simulink model "gm_VSD_and_Park_transformation_6Phase"  (R2022a)
settings: Solver=FixedStepDiscrete  StartTime=0.0  StopTime=0.2  RelTol=1e-3
libraries: hdlmdlgenlib x2
(part 1 of 2)
settings Model: Creator=Andre Merx  LastModifiedBy=Andre Merx
settings SolverCC: AlgebraicLoopSolver=TrustRegion
settings DataIOCC: LimitDataPoints=on  SaveOutput=off  SaveTime=off
settings OptimizationCC: BlockReduction=off  ConditionallyExecuteInputs=off  DefaultParameterBehavior=Inlined  InheritOutputTypeSmallerThanSingle=on  LifeSpan=inf
settings DebuggingCC: AlgebraicLoopMsg=error  InheritedTsInSrcMsg=none  SingleTaskRateTransMsg=error  UnconnectedInputMsg=warning  UnconnectedOutputMsg=warning  UnconnectedLineMsg=warning  AllowSymbolicDim=off  StrictBusMsg=ErrorOnBusTreatedAsVector  SFUnexpectedBacktrackingDiag=warning  SFNoUnconditionalDefaultTransitionDiag=warning  SFExecutionAtInitializationDiag=none  SFMachineParentedDataDiag=warning  ArithmeticOperatorsInVariantConditions=warning
settings HardwareCC: ProdBitPerPointer=32  ProdBitPerSizeT=32  ProdBitPerPtrDiffT=32  ProdLargestAtomicFloat=None  ProdIntDivRoundTo=Undefined  ProdEndianess=Unspecified  ProdWordSize=32  ProdHWDeviceType=ASIC/FPGA->ASIC/FPGA  ProdEqTarget=off
settings SFSimCC: SimUseLocalCustomCode=off  CustomCodeUndefinedFunction=UseInterfaceOnly
settings RTWCC: RTWUseLocalCustomCode=off
settings CodeAppCC: StateflowObjectComments=on
settings GRTTargetCC: TargetLangStandard=C89/C90 (ANSI)
settings ConfigComp: CovScope=ReferencedModels  CovMetricSettings=dw  CovSaveCumulativeToWorkspaceVar=on  CovSaveSingleToWorkspaceVar=on  CovExternalEMLEnable=off  CovSFcnEnable=off

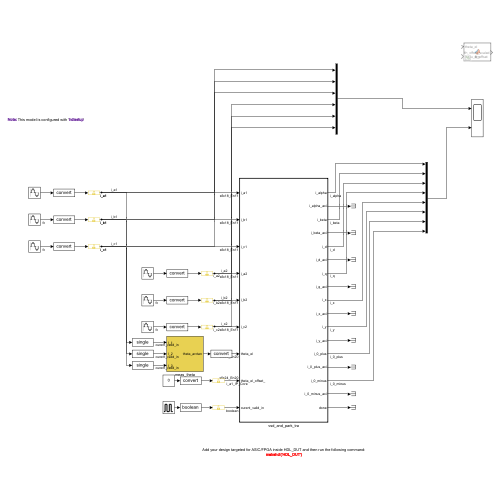
[thumbnail: Simulink's stored preview of the top-level diagram]
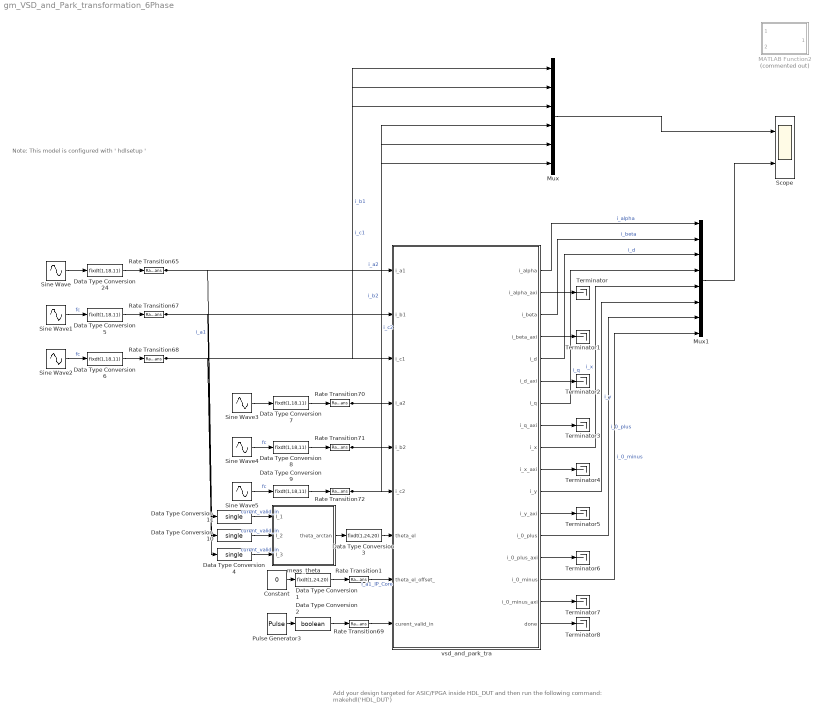
== system gm_VSD_and_Park_transformation_6Phase ==
  note: Add your design targeted for ASIC/FPGA inside HDL_DUT and then run the following command:
      | makehdl('HDL_DUT')
  note: Note: This model is configured with ' hdlsetup '
  Constant : Constant  Value=0  SampleTime=-1
  Data Type Conversion1 : DataTypeConversion  OutDataTypeStr=fixdt(1,24,20)  SaturateOnIntegerOverflow=off  RndMeth=Floor
  Data Type Conversion10 : DataTypeConversion  OutDataTypeStr=single  SaturateOnIntegerOverflow=off  RndMeth=Floor
  Data Type Conversion11 : DataTypeConversion  OutDataTypeStr=single  SaturateOnIntegerOverflow=off  RndMeth=Floor
  Data Type Conversion2 : DataTypeConversion  OutDataTypeStr=boolean  SaturateOnIntegerOverflow=off  RndMeth=Floor
  Data Type Conversion{5..9,24} (6 alike) : DataTypeConversion  OutDataTypeStr=fixdt(1,18,11)  SaturateOnIntegerOverflow=off  RndMeth=Floor
  Data Type Conversion3 : DataTypeConversion  OutDataTypeStr=fixdt(1,24,20)  SaturateOnIntegerOverflow=off  RndMeth=Floor
  Data Type Conversion4 : DataTypeConversion  OutDataTypeStr=single  SaturateOnIntegerOverflow=off  RndMeth=Floor
  MATLAB Function2 : MATLAB Function  Commented=on  TreatAsAtomicUnit=on
  Mux : Mux  Inputs=6
  Mux1 : Mux  Inputs=8
  Pulse Generator3 : DiscretePulseGenerator  PulseType=Time based  Period=1/100000  PulseWidth=5
  Rate Transition{1,65,67..72} (8 alike) : RateTransition  OutPortSampleTime=1.0000e-08
  Scope : Scope  NumInputPorts=2
  Sine Wave : Sin  Frequency=100  SampleTime=1/100000
  Sine Wave1 : Sin  Frequency=100  Phase=(4/3)*pi  SampleTime=1/100000
  Sine Wave2 : Sin  Frequency=100  Phase=(2/3)*pi  SampleTime=1/100000
  Sine Wave3 : Sin  Amplitude=0.5  Frequency=100  Phase=-pi/6  SampleTime=1/100000
  Sine Wave4 : Sin  Amplitude=0.5  Frequency=100  Phase=(7/6)*pi  SampleTime=1/100000
  Sine Wave5 : Sin  Amplitude=0.5  Frequency=100  Phase=(1/2)*pi  SampleTime=1/100000
  Terminator{,1..8} (9 alike) : Terminator
  meas_theta : Subsystem
  vsd_and_park_tra : Subsystem  TreatAsAtomicUnit=on
  wires:
  Data Type Conversion11/1 -> meas_theta/1(I_1)  "curent_valid_in"
  Data Type Conversion10/1 -> meas_theta/2(I_2)  "curent_valid_in"
  Data Type Conversion4/1 -> meas_theta/3(I_3)  "curent_valid_in"
  Data Type Conversion3/1 -> vsd_and_park_tra/7(theta_el)
  Mux1/1 -> Scope/2
  vsd_and_park_tra/15(i_0_minus) -> Mux1/8  "i_0_minus"
  vsd_and_park_tra/13(i_0_plus) -> Mux1/7  "i_0_plus"
  vsd_and_park_tra/11(i_y) -> Mux1/6  "i_y"
  vsd_and_park_tra/9(i_x) -> Mux1/5  "i_x"
  vsd_and_park_tra/7(i_q) -> Mux1/4  "i_q"
  vsd_and_park_tra/5(i_d) -> Mux1/3  "i_d"
  vsd_and_park_tra/3(i_beta) -> Mux1/2  "i_beta"
  vsd_and_park_tra/1(i_alpha) -> Mux1/1  "i_alpha"
  Mux/1 -> Scope/1
  vsd_and_park_tra/17(done) -> Terminator8/1
  vsd_and_park_tra/16(i_0_minus_axi) -> Terminator7/1
  vsd_and_park_tra/14(i_0_plus_axi) -> Terminator6/1
  vsd_and_park_tra/12(i_y_axi) -> Terminator5/1
  vsd_and_park_tra/10(i_x_axi) -> Terminator4/1
  vsd_and_park_tra/8(i_q_axi) -> Terminator3/1
  vsd_and_park_tra/6(i_d_axi) -> Terminator2/1
  vsd_and_park_tra/4(i_beta_axi) -> Terminator1/1
  vsd_and_park_tra/2(i_alpha_axi) -> Terminator/1
  Data Type Conversion2/1 -> Rate Transition69/1
  Rate Transition69/1 -> vsd_and_park_tra/9(curent_valid_in)
  Pulse Generator3/1 -> Data Type Conversion2/1
  Rate Transition1/1 -> vsd_and_park_tra/8(theta_el_offset_)  "i_a1_IP_Core"
  Data Type Conversion1/1 -> Rate Transition1/1
  Constant/1 -> Data Type Conversion1/1
  meas_theta/1(theta_arctan) -> Data Type Conversion3/1
  Rate Transition72/1 -> vsd_and_park_tra/6(i_c2), Mux/6  "i_c2"
  Rate Transition71/1 -> vsd_and_park_tra/5(i_b2), Mux/5  "i_b2"
  Rate Transition70/1 -> vsd_and_park_tra/4(i_a2), Mux/4  "i_a2"
  Data Type Conversion8/1 -> Rate Transition71/1
  Data Type Conversion7/1 -> Rate Transition70/1
  Sine Wave3/1 -> Data Type Conversion7/1
  Sine Wave4/1 -> Data Type Conversion8/1  "fc"
  Data Type Conversion9/1 -> Rate Transition72/1
  Sine Wave5/1 -> Data Type Conversion9/1  "fc"
  Rate Transition68/1 -> Data Type Conversion4/1, vsd_and_park_tra/3(i_c1), Mux/3  "i_c1"
  Rate Transition67/1 -> Data Type Conversion10/1, vsd_and_park_tra/2(i_b1), Mux/2  "i_b1"
  Rate Transition65/1 -> Data Type Conversion11/1, vsd_and_park_tra/1(i_a1), Mux/1  "i_a1"
  Data Type Conversion24/1 -> Rate Transition65/1
  Data Type Conversion5/1 -> Rate Transition67/1
  Sine Wave2/1 -> Data Type Conversion6/1  "fc"
  Data Type Conversion6/1 -> Rate Transition68/1
  Sine Wave1/1 -> Data Type Conversion5/1  "fc"
  Sine Wave/1 -> Data Type Conversion24/1

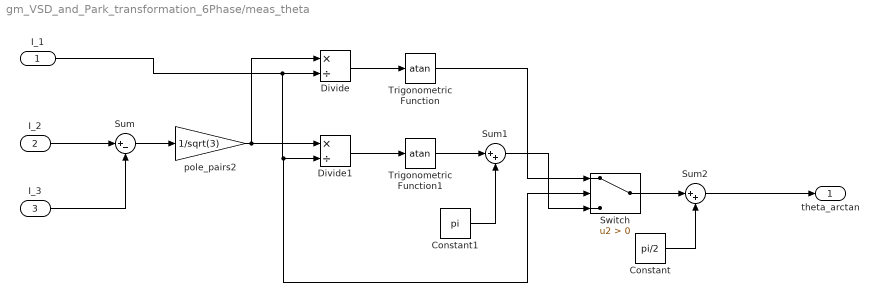
== system gm_VSD_and_Park_transformation_6Phase/meas_theta ==
  I_1 : Inport
  I_2 : Inport  Port=2
  I_3 : Inport  Port=3
  Constant : Constant  Value=pi/2
  Constant1 : Constant  Value=pi
  Divide : Product  Inputs=*/
  Divide1 : Product  Inputs=*/
  Sum : Sum  Inputs=|+-
  Sum1 : Sum  Inputs=|++
  Sum2 : Sum  Inputs=|++
  Switch : Switch  Criteria=u2 > Threshold  SaturateOnIntegerOverflow=off  InputSameDT=off
  Trigonometric Function : Trigonometry  Operator=atan
  Trigonometric Function1 : Trigonometry  Operator=atan
  pole_pairs2 : Gain  Gain=1/sqrt(3)
  theta_arctan : Outport  VectorParamsAs1DForOutWhenUnconnected=off
  wires:
  Sum2/1 -> theta_arctan/1
  Constant1/1 -> Sum1/2
  Constant/1 -> Sum2/2
  Switch/1 -> Sum2/1
  Trigonometric Function/1 -> Switch/1
  Sum1/1 -> Switch/3
  I_1/1 -> Divide/2, Divide1/2, Switch/2
  I_2/1 -> Sum/1
  I_3/1 -> Sum/2
  Sum/1 -> pole_pairs2/1
  pole_pairs2/1 -> Divide1/1, Divide/1
  Trigonometric Function1/1 -> Sum1/1
  Divide1/1 -> Trigonometric Function1/1
  Divide/1 -> Trigonometric Function/1

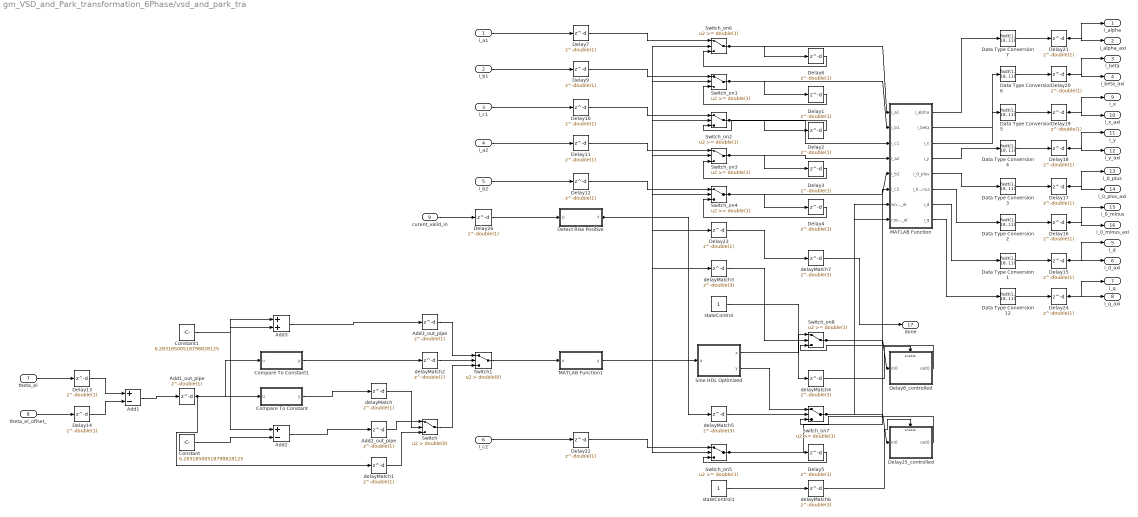
== system gm_VSD_and_Park_transformation_6Phase/vsd_and_park_tra ==
  i_a1 : Inport  OutDataTypeStr=fixdt(1, 18, 11)  PortDimensions=1  SampleTime=1e-08
  i_b1 : Inport  Port=2  OutDataTypeStr=fixdt(1, 18, 11)  PortDimensions=1  SampleTime=1e-08
  i_c1 : Inport  Port=3  OutDataTypeStr=fixdt(1, 18, 11)  PortDimensions=1  SampleTime=1e-08
  i_a2 : Inport  Port=4  OutDataTypeStr=fixdt(1, 18, 11)  PortDimensions=1  SampleTime=1e-08
  i_b2 : Inport  Port=5  OutDataTypeStr=fixdt(1, 18, 11)  PortDimensions=1  SampleTime=1e-08
  i_c2 : Inport  Port=6  OutDataTypeStr=fixdt(1, 18, 11)  PortDimensions=1  SampleTime=1e-08
  theta_el : Inport  Port=7  OutDataTypeStr=fixdt(1, 24, 20)  PortDimensions=1  SampleTime=1e-08
  theta_el_offset_ : Inport  Port=8  OutDataTypeStr=fixdt(1, 24, 20)  PortDimensions=1  SampleTime=1e-08
  curent_valid_in : Inport  Port=9  OutDataTypeStr=boolean  PortDimensions=1  SampleTime=1e-08
  Add1 : Sum  Inputs=+-  AccumDataTypeStr=fixdt(1, 24, 20)  OutDataTypeStr=fixdt(1, 24, 20)  RndMeth=Simplest  SampleTime=1e-08
  Add1_out_pipe : Delay  DelayLength=double(1)  InitialCondition=0  SampleTime=1e-08
  Add2 : Sum  Inputs=+-  AccumDataTypeStr=fixdt(1, 24, 20)  OutDataTypeStr=fixdt(1, 24, 20)  RndMeth=Simplest  SampleTime=1e-08
  Add2_out_pipe : Delay  DelayLength=double(1)  InitialCondition=0  SampleTime=1e-08
  Add3 : Sum  AccumDataTypeStr=fixdt(1, 24, 20)  OutDataTypeStr=fixdt(1, 24, 20)  RndMeth=Simplest  SampleTime=1e-08
  Add3_out_pipe : Delay  DelayLength=double(1)  InitialCondition=0  SampleTime=1e-08
  Compare To Constant : Subsystem  mask(Compare To Constant){relop=>=, const=double(6.283185307179586), OutDataTypeStr=boolean, ZeroCross=on}
      mask prompts: relop "Simulink:masks:Operator_MP"; const "Simulink:masks:ConstantValue_MP"; OutDataTypeStr "Simulink:masks:OutputDataType_MP"; ZeroCross "Simulink:masks:EnableZerocrossingDetection_MP"
      mask help: Simulink:masks:CompareToConstant_MD
      mask init:
      | OutDataTypeStr = 'boolean';
      | ZeroCross = 'on';
      | blkName = 'VSD_and_Park_transformation_6Phase/vsd_and_park_tra/Compare\nTo Constant';
      | const = double(6.283185307179586);
      | const_str = '2*pi';
      | const_val = double(6.283185307179586);
      | relop = '>=';
      | setValue = 'boolean';
      | str = '>= 6.2832';
      mask TypeOptions relop: == | ~= | < | <= | >= | >
      mask TypeOptions OutDataTypeStr: Simulink:masks:uint8 | Simulink:masks:boolean
      mask Callback ZeroCross: sl('zeroCrossEnable', gcbh);
      mask Display: disp(str)
  Compare To Constant1 : Subsystem  mask(Compare To Constant){relop=<, const=double(0), OutDataTypeStr=boolean, ZeroCross=on}
      mask prompts: relop "Simulink:masks:Operator_MP"; const "Simulink:masks:ConstantValue_MP"; OutDataTypeStr "Simulink:masks:OutputDataType_MP"; ZeroCross "Simulink:masks:EnableZerocrossingDetection_MP"
      mask help: Simulink:masks:CompareToConstant_MD
      mask init:
      | OutDataTypeStr = 'boolean';
      | ZeroCross = 'on';
      | blkName = 'VSD_and_Park_transformation_6Phase/vsd_and_park_tra/Compare\nTo Constant1';
      | const = double(0);
      | const_str = '0';
      | const_val = double(0);
      | relop = '<';
      | setValue = 'boolean';
      | str = '< 0';
      mask TypeOptions relop: == | ~= | < | <= | >= | >
      mask TypeOptions OutDataTypeStr: Simulink:masks:uint8 | Simulink:masks:boolean
      mask Callback ZeroCross: sl('zeroCrossEnable', gcbh);
      mask Display: disp(str)
  Constant : Constant  Value=6.28318500518798828125  OutDataTypeStr=fixdt(1, 24, 20)  SampleTime=1e-08
  Constant1 : Constant  Value=6.28318500518798828125  OutDataTypeStr=fixdt(1, 24, 20)  SampleTime=1e-08
  Data Type Conversion{1..7,12} (8 alike) : DataTypeConversion  OutDataTypeStr=fixdt(1, 18, 11)  RndMeth=Simplest  SampleTime=1e-08  SaturateOnIntegerOverflow=off
  Delay{1..7,9..24,26} (24 alike) : Delay  DelayLength=double(1)  InitialCondition=0  SampleTime=1e-08
  Delay25_controlled : Subsystem
  Delay8_controlled : Subsystem
  Detect Rise Positive : Subsystem  mask(Detect Rise Positive){vinit=double(0), InputProcessing=Elements as channels (sample based), OutDataTypeStr=boolean}
      mask prompts: vinit "Simulink:masks:InitialCondition_MP"; InputProcessing "Simulink:masks:InputProcessing_MP"; OutDataTypeStr "Simulink:masks:OutputDataType_MP"
      mask help: Simulink:masks:DetectRisePositive_MD
      mask init:
      | InputProcessing = 'Elements as channels (sample based)';
      | OutDataTypeStr = 'boolean';
      | vinit = double(0);
      mask TypeOptions InputProcessing: Simulink:masks:ColumnsAsChannelsFrameBased | Simulink:masks:ElementsAsChannelsSampleBased
      mask TypeOptions OutDataTypeStr: Simulink:masks:uint8 | Simulink:masks:boolean
      mask Display: fprintf('U > 0\n&  NOT\nU/z > 0')
  MATLAB Function : Subsystem
  MATLAB Function1 : Subsystem
  Sine HDL Optimized : Subsystem  mask(Sine and Cosine HDL optimized block){OutputFormula=sin(2*pi*u) and cos(2*pi*u), NumDataPoints=double(512), TableDataTypeStr=fixdt(1,17,11), SimulateLUTROMDelay=off}
      mask prompts: OutputFormula "Simulink:masks:OutputFormula_MP"; NumDataPoints "HDLShared:hdlshared:CosineHDL_Npts"; TableDataTypeStr "Simulink:blkprm_prompts:TABLE_UNIFIEDDATATYPE"; SimulateLUTROMDelay "HDLShared:hdlshared:CosineHDL_SimulateLUTDelay"
      mask help: Sine and Cosine HDL optimized block using quarter wave symmetry, and HDL friendly settings.
      mask Help: helpview([docroot '/hdlcoder/helptargets.map'],'SineAndCosineHDL_Optimized');
      mask TypeOptions OutputFormula: sin(2*pi*u) | cos(2*pi*u) | exp(j*2*pi*u) | sin(2*pi*u) and cos(2*pi*u)
      mask Display:
      | port_label('input',1,'u')
      | port_label('output',1,'sin(2*pi*u)')
      | port_label('output',2,'cos(2*pi*u)')
      | xpos = 0.35;
      | yoffset = 0.5;
      | if ( SimulateLUTROMDelay )
      |   text(xpos,yoffset,'HDL (Z^{-1})','texmode','on')
      | else
      |    text(xpos,yoffset,'HDL')
      | end
  Switch : Switch  Criteria=u2 > Threshold  Threshold=double(0)  OutDataTypeStr=fixdt(1, 24, 20)  RndMeth=Simplest  SampleTime=1e-08  SaturateOnIntegerOverflow=off  InputSameDT=off
  Switch1 : Switch  Criteria=u2 > Threshold  Threshold=double(0)  OutDataTypeStr=fixdt(1, 24, 20)  RndMeth=Simplest  SampleTime=1e-08  SaturateOnIntegerOverflow=off  InputSameDT=off
  Switch_on{1..8} (8 alike) : Switch  Threshold=double(1)  OutDataTypeStr=fixdt(1, 18, 11)  RndMeth=Simplest  SampleTime=1e-08  SaturateOnIntegerOverflow=off  InputSameDT=off
  delayMatch : Delay  DelayLength=double(1)  InitialCondition=0  SampleTime=1e-08
  delayMatch1 : Delay  DelayLength=double(1)  InitialCondition=0  SampleTime=1e-08
  delayMatch2 : Delay  DelayLength=double(1)  InitialCondition=0  SampleTime=1e-08
  delayMatch{3..7} (5 alike) : Delay  DelayLength=double(3)  InitialCondition=0  SampleTime=1e-08
  stateControl : Constant  OutDataTypeStr=boolean  SampleTime=1e-08
  stateControl1 : Constant  OutDataTypeStr=boolean  SampleTime=1e-08
  i_alpha : Outport  SampleTime=1e-08
  i_alpha_axi : Outport  Port=2  SampleTime=1e-08
  i_beta : Outport  Port=3  SampleTime=1e-08
  i_beta_axi : Outport  Port=4  SampleTime=1e-08
  i_d : Outport  Port=5  SampleTime=1e-08
  i_d_axi : Outport  Port=6  SampleTime=1e-08
  i_q : Outport  Port=7  SampleTime=1e-08
  i_q_axi : Outport  Port=8  SampleTime=1e-08
  i_x : Outport  Port=9  SampleTime=1e-08
  i_x_axi : Outport  Port=10  SampleTime=1e-08
  i_y : Outport  Port=11  SampleTime=1e-08
  i_y_axi : Outport  Port=12  SampleTime=1e-08
  i_0_plus : Outport  Port=13  SampleTime=1e-08
  i_0_plus_axi : Outport  Port=14  SampleTime=1e-08
  i_0_minus : Outport  Port=15  SampleTime=1e-08
  i_0_minus_axi : Outport  Port=16  SampleTime=1e-08
  done : Outport  Port=17  SampleTime=1e-08
  wires:
  i_a1/1 -> Delay7/1
  i_b1/1 -> Delay9/1
  i_c1/1 -> Delay10/1
  i_a2/1 -> Delay11/1
  i_b2/1 -> Delay12/1
  i_c2/1 -> Delay22/1
  theta_el/1 -> Delay13/1
  theta_el_offset_/1 -> Delay14/1
  curent_valid_in/1 -> Delay26/1
  delayMatch1/1 -> Switch/3
  Add2_out_pipe/1 -> Switch/1
  Add3_out_pipe/1 -> Switch1/1
  delayMatch/1 -> Switch/2
  delayMatch2/1 -> Switch1/2
  Constant/1 -> Add2/2
  Constant1/1 -> Add3/2
  Data Type Conversion1/1 -> Delay15/1
  Data Type Conversion12/1 -> Delay24/1
  Data Type Conversion2/1 -> Delay16/1
  Data Type Conversion3/1 -> Delay17/1
  Data Type Conversion4/1 -> Delay18/1
  Data Type Conversion5/1 -> Delay19/1
  Data Type Conversion6/1 -> Delay20/1
  Data Type Conversion7/1 -> Delay21/1
  Delay10/1 -> Switch_on2/1
  Delay11/1 -> Switch_on3/1
  Delay12/1 -> Switch_on4/1
  Delay13/1 -> Add1/1
  Delay14/1 -> Add1/2
  Delay15/1 -> i_d_axi/1, i_d/1
  Delay16/1 -> i_0_minus_axi/1, i_0_minus/1
  Delay17/1 -> i_0_plus_axi/1, i_0_plus/1
  Delay18/1 -> i_y_axi/1, i_y/1
  Delay19/1 -> i_x_axi/1, i_x/1
  Delay20/1 -> i_beta_axi/1, i_beta/1
  Delay21/1 -> i_alpha_axi/1, i_alpha/1
  Delay22/1 -> Switch_on5/1
  delayMatch7/1 -> done/1
  Delay24/1 -> i_q_axi/1, i_q/1
  Delay26/1 -> Detect Rise Positive/1(U)
  Delay7/1 -> Switch_on6/1
  Delay9/1 -> Switch_on1/1
  delayMatch3/1 -> Switch_on8/2
  MATLAB Function/1(i_alpha) -> Data Type Conversion7/1
  MATLAB Function/2(i_beta) -> Data Type Conversion6/1
  MATLAB Function/3(i_x) -> Data Type Conversion5/1
  MATLAB Function/4(i_y) -> Data Type Conversion4/1
  MATLAB Function/5(i_0_plus) -> Data Type Conversion3/1
  MATLAB Function/6(i_0_minus) -> Data Type Conversion2/1
  MATLAB Function/7(i_d) -> Data Type Conversion1/1
  MATLAB Function/8(i_q) -> Data Type Conversion12/1
  MATLAB Function1/1(y) -> Sine HDL Optimized/1(u)
  Sine HDL Optimized/1(x) -> Switch_on8/1
  Sine HDL Optimized/2(y) -> Switch_on7/1
  Switch/1 -> Switch1/3
  Switch1/1 -> MATLAB Function1/1(u)
  Switch_on1/1 -> MATLAB Function/2(i_b1), Delay1/1
  Switch_on2/1 -> MATLAB Function/3(i_c1), Delay2/1
  Switch_on3/1 -> MATLAB Function/4(i_a2), Delay3/1
  Switch_on4/1 -> MATLAB Function/5(i_b2), Delay4/1
  Switch_on5/1 -> MATLAB Function/6(i_c2), Delay5/1
  Switch_on6/1 -> MATLAB Function/1(i_a1), Delay6/1
  Add1/1 -> Add1_out_pipe/1
  Add2/1 -> Add2_out_pipe/1
  Add3/1 -> Add3_out_pipe/1
  delayMatch4/1 -> Delay8_controlled/Enable
  delayMatch6/1 -> Delay25_controlled/Enable
  Compare To Constant/1(y) -> delayMatch/1
  Add1_out_pipe/1 -> delayMatch1/1, Add3/1, Add2/1, Compare To Constant1/1(u), Compare To Constant/1(u)
  Compare To Constant1/1(y) -> delayMatch2/1
  delayMatch5/1 -> Switch_on7/2
  stateControl/1 -> delayMatch4/1
  Detect Rise Positive/1(Y) -> delayMatch5/1, delayMatch3/1, Delay23/1, Switch_on6/2, Switch_on1/2, Switch_on2/2, Switch_on3/2, Switch_on4/2, Switch_on5/2
  stateControl1/1 -> delayMatch6/1
  Delay23/1 -> delayMatch7/1
  Delay6/1 -> Switch_on6/3
  Delay1/1 -> Switch_on1/3
  Delay2/1 -> Switch_on2/3
  Delay3/1 -> Switch_on3/3
  Delay4/1 -> Switch_on4/3
  Delay5/1 -> Switch_on5/3
  Delay8_controlled/1(out0) -> Switch_on8/3
  Switch_on8/1 -> Delay8_controlled/1(in0), MATLAB Function/7(sin_theta_el)
  Delay25_controlled/1(out0) -> Switch_on7/3
  Switch_on7/1 -> Delay25_controlled/1(in0), MATLAB Function/8(cos_theta_el)

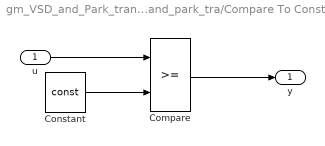
== system gm_VSD_and_Park_transformation_6Phase/vsd_and_park_tra/Compare To Constant ==
  u : Inport  OutDataTypeStr=fixdt(1, 24, 20)  SampleTime=1e-08
  Compare : RelationalOperator  OutDataTypeStr=boolean
  Constant : Constant  DisableCoverage=on  Value=const  OutDataTypeStr=Inherit: Inherit via back propagation  SampleTime=-1
  y : Outport  SampleTime=1e-08
  wires:
  Compare/1 -> y/1
  Constant/1 -> Compare/2
  u/1 -> Compare/1

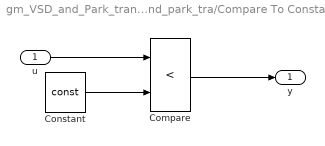
== system gm_VSD_and_Park_transformation_6Phase/vsd_and_park_tra/Compare To Constant1 ==
  u : Inport  OutDataTypeStr=fixdt(1, 24, 20)  SampleTime=1e-08
  Compare : RelationalOperator  Operator=<  OutDataTypeStr=boolean
  Constant : Constant  DisableCoverage=on  Value=const  OutDataTypeStr=Inherit: Inherit via back propagation  SampleTime=-1
  y : Outport  SampleTime=1e-08
  wires:
  Compare/1 -> y/1
  Constant/1 -> Compare/2
  u/1 -> Compare/1

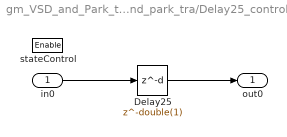
== system gm_VSD_and_Park_transformation_6Phase/vsd_and_park_tra/Delay25_controlled ==
  in0 : Inport  OutDataTypeStr=fixdt(1, 18, 11)  SampleTime=1e-08
  stateControl : EnablePort  OutDataTypeStr=boolean
  Delay25 : Delay  DelayLength=double(1)  InitialCondition=0  SampleTime=1e-08
  out0 : Outport  OutDataTypeStr=fixdt(1, 18, 11)  SampleTime=1e-08
  wires:
  Delay25/1 -> out0/1
  in0/1 -> Delay25/1

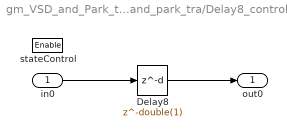
== system gm_VSD_and_Park_transformation_6Phase/vsd_and_park_tra/Delay8_controlled ==
  in0 : Inport  OutDataTypeStr=fixdt(1, 18, 11)  SampleTime=1e-08
  stateControl : EnablePort  OutDataTypeStr=boolean
  Delay8 : Delay  DelayLength=double(1)  InitialCondition=0  SampleTime=1e-08
  out0 : Outport  OutDataTypeStr=fixdt(1, 18, 11)  SampleTime=1e-08
  wires:
  Delay8/1 -> out0/1
  in0/1 -> Delay8/1

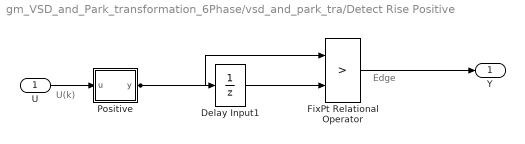
== system gm_VSD_and_Park_transformation_6Phase/vsd_and_park_tra/Detect Rise Positive ==
  note: Edge
  note: U(k)
  U : Inport  OutDataTypeStr=boolean  SampleTime=1e-08
  Delay Input1 : UnitDelay  Description=Store in Global RAM  DisableCoverage=on  InitialCondition=vinit  SampleTime=-1  HasFrameUpgradeWarning=on
  FixPt Relational Operator : RelationalOperator  Operator=>  OutDataTypeStr=boolean  ZeroCross=off  InputSameDT=off
  Positive : Subsystem  mask(Compare To Zero){relop=>, OutDataTypeStr=boolean, ZeroCross=off}
      mask prompts: relop "Simulink:masks:Operator_MP"; OutDataTypeStr "Simulink:masks:OutputDataType_MP"; ZeroCross "Simulink:masks:EnableZerocrossingDetection_MP"
      mask help: Simulink:masks:CompareToZero_MD
      mask init:
      | OutDataTypeStr = 'boolean';
      | ZeroCross = 'off';
      | blkName = 'VSD_and_Park_transformation_6Phase/vsd_and_park_tra/Detect Rise\nPositive/Positive';
      | relop = '>';
      | setValue = 'boolean';
      mask TypeOptions relop: == | ~= | < | <= | >= | >
      mask TypeOptions OutDataTypeStr: Simulink:masks:uint8 | Simulink:masks:boolean
      mask Callback ZeroCross: sl('zeroCrossEnable', gcbh);
      mask Display: disp([relop,' 0'])
  Y : Outport  SampleTime=1e-08
  wires:
  Delay Input1/1 -> FixPt Relational Operator/2
  FixPt Relational Operator/1 -> Y/1
  Positive/1(y) -> FixPt Relational Operator/1, Delay Input1/1
  U/1 -> Positive/1(u)

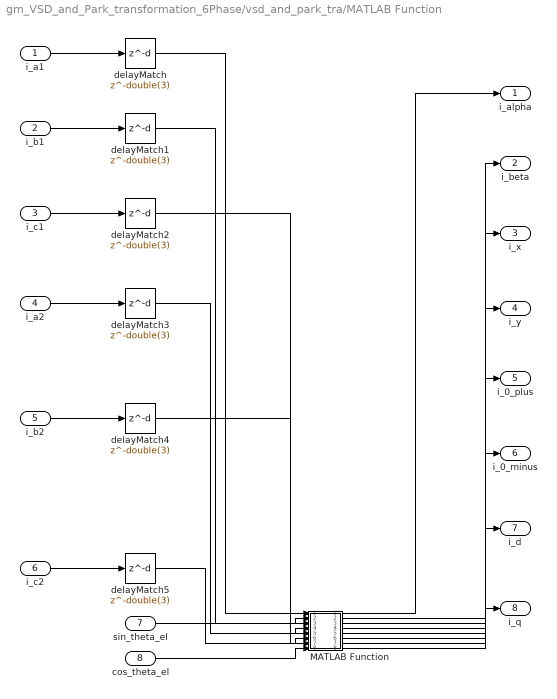
== system gm_VSD_and_Park_transformation_6Phase/vsd_and_park_tra/MATLAB Function ==
  i_a1 : Inport  OutDataTypeStr=fixdt(1, 18, 11)  PortDimensions=1  SampleTime=1e-08
  i_b1 : Inport  Port=2  OutDataTypeStr=fixdt(1, 18, 11)  PortDimensions=1  SampleTime=1e-08
  i_c1 : Inport  Port=3  OutDataTypeStr=fixdt(1, 18, 11)  PortDimensions=1  SampleTime=1e-08
  i_a2 : Inport  Port=4  OutDataTypeStr=fixdt(1, 18, 11)  PortDimensions=1  SampleTime=1e-08
  i_b2 : Inport  Port=5  OutDataTypeStr=fixdt(1, 18, 11)  PortDimensions=1  SampleTime=1e-08
  i_c2 : Inport  Port=6  OutDataTypeStr=fixdt(1, 18, 11)  PortDimensions=1  SampleTime=1e-08
  sin_theta_el : Inport  Port=7  OutDataTypeStr=fixdt(1, 18, 11)  PortDimensions=1  SampleTime=1e-08
  cos_theta_el : Inport  Port=8  OutDataTypeStr=fixdt(1, 18, 11)  PortDimensions=1  SampleTime=1e-08
  MATLAB Function : MATLAB Function  TreatAsAtomicUnit=on
  delayMatch{,1..5} (6 alike) : Delay  DelayLength=double(3)  InitialCondition=0  SampleTime=1e-08
  i_alpha : Outport  SampleTime=1e-08  VectorParamsAs1DForOutWhenUnconnected=off
  i_beta : Outport  Port=2  SampleTime=1e-08
  i_x : Outport  Port=3  SampleTime=1e-08
  i_y : Outport  Port=4  SampleTime=1e-08
  i_0_plus : Outport  Port=5  SampleTime=1e-08
  i_0_minus : Outport  Port=6  SampleTime=1e-08
  i_d : Outport  Port=7  SampleTime=1e-08
  i_q : Outport  Port=8  SampleTime=1e-08
  wires:
  delayMatch/1 -> MATLAB Function/1(i_a1)
  delayMatch1/1 -> MATLAB Function/2(i_b1)
  delayMatch2/1 -> MATLAB Function/3(i_c1)
  delayMatch3/1 -> MATLAB Function/4(i_a2)
  delayMatch4/1 -> MATLAB Function/5(i_b2)
  delayMatch5/1 -> MATLAB Function/6(i_c2)
  MATLAB Function/1(i_alpha) -> i_alpha/1
  MATLAB Function/2(i_beta) -> i_beta/1
  MATLAB Function/3(i_x) -> i_x/1
  MATLAB Function/4(i_y) -> i_y/1
  MATLAB Function/5(i_0_plus) -> i_0_plus/1
  MATLAB Function/6(i_0_minus) -> i_0_minus/1
  MATLAB Function/7(i_d) -> i_d/1
  MATLAB Function/8(i_q) -> i_q/1
  i_a1/1 -> delayMatch/1
  i_b1/1 -> delayMatch1/1
  i_c1/1 -> delayMatch2/1
  i_a2/1 -> delayMatch3/1
  i_b2/1 -> delayMatch4/1
  i_c2/1 -> delayMatch5/1
  sin_theta_el/1 -> MATLAB Function/7(sin_theta_el)
  cos_theta_el/1 -> MATLAB Function/8(cos_theta_el)

== system gm_VSD_and_Park_transformation_6Phase/vsd_and_park_tra/MATLAB Function1 ==
  u : Inport  OutDataTypeStr=fixdt(1, 24, 20)  PortDimensions=1  SampleTime=1e-08
  MATLAB Function1 : MATLAB Function  TreatAsAtomicUnit=on
  y : Outport  SampleTime=1e-08  VectorParamsAs1DForOutWhenUnconnected=off
  wires:
  MATLAB Function1/1(y) -> y/1
  u/1 -> MATLAB Function1/1(u)

== system gm_VSD_and_Park_transformation_6Phase/vsd_and_park_tra/Sine HDL Optimized ==
  u : Inport  OutDataTypeStr=fixdt(1, 48, 45)  SampleTime=1e-08
  sincos hdl : Subsystem  mask{NumDataPoints=512, TableDataTypeStr=fixdt(1,17,11), SimulateLUTROMDelay='Off'}
      mask prompts: NumDataPoints "HDLShared:hdlshared:CosineHDL_Npts"; TableDataTypeStr "Simulink:blkprm_prompts:TABLE_UNIFIEDDATATYPE"; SimulateLUTROMDelay "HDLShared:hdlshared:CosineHDL_SimulateLUTDelay"
      mask Display:
      | port_label('input',1,'u')
      | port_label('output',1,'sin(2*pi*u)')
      | port_label('output',2,'cos(2*pi*u)')
      | xpos = 0.35;
      | yoffset = 0.5;
      | if ( SimulateLUTROMDelay )
      |   text(xpos,yoffset,'HDL (Z^{-1})','texmode','on')
      | else
      |    text(xpos,yoffset,'HDL')
      | end
  x : Outport  SampleTime=1e-08
  y : Outport  Port=2  SampleTime=1e-08
  wires:
  sincos hdl/1(Out1) -> x/1
  sincos hdl/2(Out2) -> y/1
  u/1 -> sincos hdl/1(In1)

== system gm_VSD_and_Park_transformation_6Phase/vsd_and_park_tra/Detect Rise Positive/Positive ==
  u : Inport  OutDataTypeStr=boolean  SampleTime=1e-08
  Compare : RelationalOperator  Operator=>  OutDataTypeStr=boolean  ZeroCross=off
  Constant : Constant  DisableCoverage=on  Value=0  OutDataTypeStr=Inherit: Inherit via back propagation  SampleTime=-1  PreserveConstantTs=on
  y : Outport  SampleTime=1e-08
  wires:
  Compare/1 -> y/1
  Constant/1 -> Compare/2
  u/1 -> Compare/1

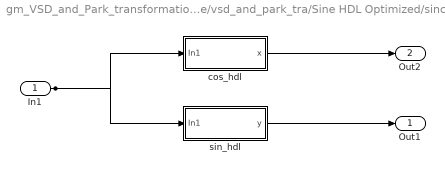
== system gm_VSD_and_Park_transformation_6Phase/vsd_and_park_tra/Sine HDL Optimized/sincos hdl ==
  In1 : Inport  OutDataTypeStr=fixdt(1, 48, 45)  SampleTime=1e-08
  cos_hdl : Subsystem  mask{NumDataPoints=double(512), TableDataTypeStr=fixdt(1,17,11), SimulateLUTROMDelay=Off}
      mask prompts: NumDataPoints "HDLShared:hdlshared:CosineHDL_Npts"; TableDataTypeStr "Simulink:blkprm_prompts:TABLE_UNIFIEDDATATYPE"; SimulateLUTROMDelay "HDLShared:hdlshared:CosineHDL_SimulateLUTDelay"
      mask Display:
      | port_label('input',1,'u')
      | port_label('output',1,'cos(2*pi*u)')
      | xpos = 0.35;
      | yoffset = 0.5;
      | if ( SimulateLUTROMDelay )
      |   text(xpos,yoffset,'HDL (Z^{-1})','texmode','on')
      | else
      |    text(xpos,yoffset,'HDL')
      | end
  sin_hdl : Subsystem  mask{NumDataPoints=double(512), TableDataTypeStr=fixdt(1,17,11), SimulateLUTROMDelay=Off}
      mask prompts: NumDataPoints "HDLShared:hdlshared:CosineHDL_Npts"; TableDataTypeStr "Simulink:blkprm_prompts:TABLE_UNIFIEDDATATYPE"; SimulateLUTROMDelay "HDLShared:hdlshared:CosineHDL_SimulateLUTDelay"
      mask Display:
      | port_label('input',1,'u')
      | port_label('output',1,'sin(2*pi*u)')
      | xpos = 0.35;
      | yoffset = 0.5;
      | if ( SimulateLUTROMDelay )
      |   text(xpos,yoffset,'HDL (Z^{-1})','texmode','on')
      | else
      |    text(xpos,yoffset,'HDL')
      | end
  Out1 : Outport  SampleTime=1e-08
  Out2 : Outport  Port=2  SampleTime=1e-08
  wires:
  cos_hdl/1(x) -> Out2/1
  sin_hdl/1(y) -> Out1/1
  In1/1 -> cos_hdl/1(In1), sin_hdl/1(In1)

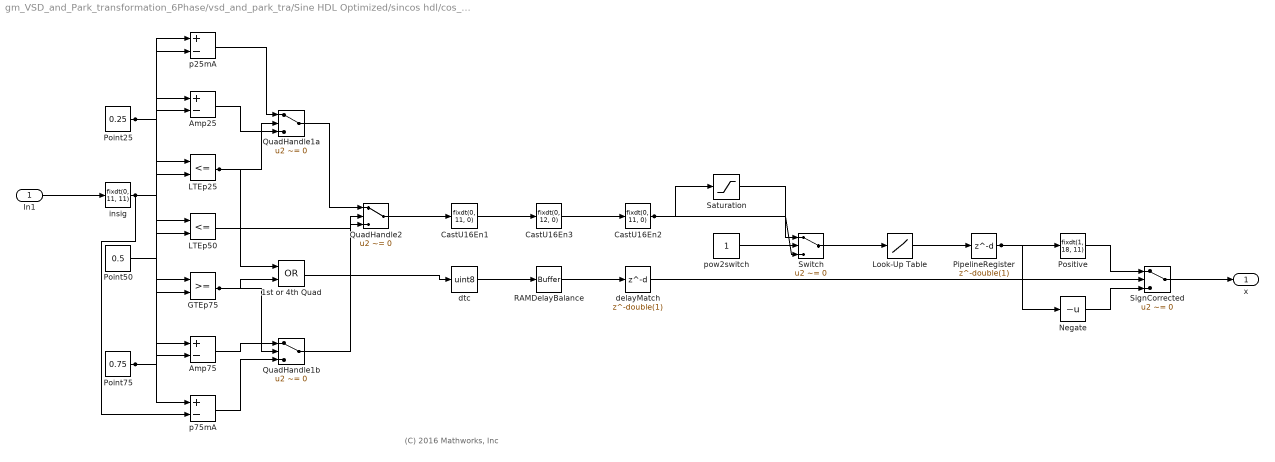
== system gm_VSD_and_Park_transformation_6Phase/vsd_and_park_tra/Sine HDL Optimized/sincos hdl/cos_hdl ==
  note: (C) 2016 Mathworks, Inc
  In1 : Inport  OutDataTypeStr=fixdt(1, 48, 45)  SampleTime=1e-08
  1st or 4th Quad : Logic  Operator=OR  AllPortsSameDT=off  OutDataTypeStr=boolean  SampleTime=1e-08
  Amp25 : Sum  Inputs=+-  AccumDataTypeStr=fixdt(1, 19, 18)  OutDataTypeStr=fixdt(1, 19, 18)  SampleTime=1e-08
  Amp75 : Sum  Inputs=+-  AccumDataTypeStr=fixdt(1, 19, 18)  OutDataTypeStr=fixdt(1, 19, 18)  SampleTime=1e-08
  CastU16En1 : DataTypeConversion  OutDataTypeStr=fixdt(0, 11, 0)  ConvertRealWorld=Stored Integer (SI)  SampleTime=1e-08  SaturateOnIntegerOverflow=off  RndMeth=Floor
  CastU16En2 : DataTypeConversion  OutDataTypeStr=fixdt(0, 11, 0)  ConvertRealWorld=Stored Integer (SI)  SampleTime=1e-08  RndMeth=Floor
  CastU16En3 : DataTypeConversion  OutDataTypeStr=fixdt(0, 12, 0)  SampleTime=1e-08  SaturateOnIntegerOverflow=off  RndMeth=Floor
  GTEp75 : RelationalOperator  OutDataTypeStr=boolean  SampleTime=1e-08  InputSameDT=off
  LTEp25 : RelationalOperator  Operator=<=  OutDataTypeStr=boolean  SampleTime=1e-08  InputSameDT=off
  LTEp50 : RelationalOperator  Operator=<=  OutDataTypeStr=boolean  SampleTime=1e-08  InputSameDT=off
  Look-Up Table : Lookup_n-D  NumberOfTableDimensions=1  BreakpointsForDimension1="fi(\"numerictype\",numerictype(0,11,0),\"fimath\",fimath(\"RoundingMethod\", \"Floor\",\"OverflowAction\", \"Wrap\",\"ProductMode\",\"FullPrecision\",\"SumMode\",\"FullPrecision\"),\"Value\",\"[0 1 2 3 4 5 6 7 8 9 10 11 12 13 14 15 16 17 18 19 20 21 22 23 24 25 26 27 28 29 30 31 32 33 34 35 36 37 38 39 40 41 42 43 44 45 46 47 48 49 50 51 52 53 54 55 56 57 58 59 60 61 62 63 64 65 66 67 68 69 70 71 72 73 74 75 76 77 78 79 80 81 82 83 84 85 86 87 88 89 90 91 92 93 94 95 96 97 98 99 100 101 102 103 104 105 106 107 108 109 110 111 112 113 114 115 116 117 118 119 120 121 122 123 124 125 126 127 128 129 130 131 132 133 134 135 136 137 138 139 140 141 142 143 144 145 146 147 148 149 150 151 152 153 154 155 156 157 158 159 160 161 162 163 164 165 166 167 168 169 170 171 172 173 174 175 176 177 178 179 180 181 182 183 184 185 186 187 188 189 190 191 192 193 194 195 196 197 198 199 200 201 202 203 204 205 206 207 208 209 210 211 212 213 214 215 216 217 218 219 220 221 222 223 224 225 226 227 228 229 230 231 232 233 234 235 236 237 238 239 240 241 242 243 244 245 246 247 248 249 250 251 252 253 254 255 256 257 258 259 260 261 262 263 264 265 266 267 268 269 270 271 272 273 274 275 276 277 278 279 280 281 282 283 284 285 286 287 288 289 290 291 292 293 294 295 296 297 298 299 300 301 302 303 304 305 306 307 308 309 310 311 312 313 314 315 316 317 318 319 320 321 322 323 324 325 326 327 328 329 330 331 332 333 334 335 336 337 338 339 340 341 342 343 344 345 346 347 348 349 350 351 352 353 354 355 356 357 358 359 360 361 362 363 364 365 366 367 368 369 370 371 372 373 374 375 376 377 378 379 380 381 382 383 384 385 386 387 388 389 390 391 392 393 394 395 396 397 398 399 400 401 402 403 404 405 406 407 408 409 410 411 412 413 414 415 416 417 418 419 420 421 422 423 424 425 426 427 428 429 430 431 432 433 434 435 436 437 438 439 440 441 442 443 444 445 446 447 448 449 450 451 452 453 454 455 456 457 458 459 460 461 462 463 464 465 466 467 468 469 470 471 472 473 474 475 476 477 478 479 480 481 482 483 484 485 486 487 488 489 490 491 492 493 494 495 496 497 498 499 500 501 502 503 504 505 506 507 508 509 510 511]\")"  Table="reshape(fi(\"numerictype\",numerictype(1,18,11),\"fimath\",fimath(\"RoundingMethod\", \"Floor\",\"OverflowAction\", \"Wrap\",\"ProductMode\",\"FullPrecision\",\"SumMode\",\"FullPrecision\"),\"Value\",\"[0;0.0029296875;0.00634765625;0.00927734375;0.01220703125;0.01513671875;0.0185546875;0.021484375;0.0244140625;0.02783203125;0.03076171875;0.03369140625;0.037109375;0.0400390625;0.04296875;0.0458984375;0.04931640625;0.05224609375;0.05517578125;0.05859375;0.0615234375;0.064453125;0.0673828125;0.07080078125;0.07373046875;0.07666015625;0.080078125;0.0830078125;0.0859375;0.0888671875;0.09228515625;0.09521484375;0.09814453125;0.10107421875;0.1044921875;0.107421875;0.1103515625;0.11328125;0.11669921875;0.11962890625;0.12255859375;0.12548828125;0.12890625;0.1318359375;0.134765625;0.1376953125;0.14111328125;0.14404296875;0.14697265625;0.14990234375;0.1533203125;0.15625;0.1591796875;0.162109375;0.1650390625;0.16845703125;0.17138671875;0.17431640625;0.17724609375;0.18017578125;0.18359375;0.1865234375;0.189453125;0.1923828125;0.1953125;0.1982421875;0.20166015625;0.20458984375;0.20751953125;0.21044921875;0.21337890625;0.21630859375;0.2197265625;0.22265625;0.2255859375;0.228515625;0.2314453125;0.234375;0.2373046875;0.240234375;0.24365234375;0.24658203125;0.24951171875;0.25244140625;0.25537109375;0.25830078125;0.26123046875;0.26416015625;0.26708984375;0.27001953125;0.27294921875;0.27587890625;0.27880859375;0.2822265625;0.28515625;0.2880859375;0.291015625;0.2939453125;0.296875;0.2998046875;0.302734375;0.3056640625;0.30859375;0.3115234375;0.314453125;0.3173828125;0.3203125;0.3232421875;0.32568359375;0.32861328125;0.33154296875;0.33447265625;0.33740234375;0.34033203125;0.34326171875;0.34619140625;0.34912109375;0.35205078125;0.35498046875;0.35791015625;0.3603515625;0.36328125;0.3662109375;0.369140625;0.3720703125;0.375;0.3779296875;0.38037109375;0.38330078125;0.38623046875;0.38916015625;0.39208984375;0.39453125;0.3974609375;0.400390625;0.4033203125;0.40576171875;0.40869140625;0.41162109375;0.41455078125;0.4169921875;0.419921875;0.4228515625;0.42578125;0.42822265625;0.43115234375;0.43408203125;0.4365234375;0.439453125;0.4423828125;0.44482421875;0.44775390625;0.4501953125;0.453125;0.4560546875;0.45849609375;0.46142578125;0.4638671875;0.466796875;0.4697265625;0.47216796875;0.47509765625;0.4775390625;0.48046875;0.48291015625;0.48583984375;0.48828125;0.4912109375;0.49365234375;0.49658203125;0.4990234375;0.501953125;0.50439453125;0.50732421875;0.509765625;0.51220703125;0.51513671875;0.517578125;0.5205078125;0.52294921875;0.525390625;0.5283203125;0.53076171875;0.533203125;0.5361328125;0.53857421875;0.541015625;0.54345703125;0.54638671875;0.548828125;0.55126953125;0.55419921875;0.556640625;0.55908203125;0.5615234375;0.56396484375;0.56689453125;0.5693359375;0.57177734375;0.57421875;0.57666015625;0.5791015625;0.58203125;0.58447265625;0.5869140625;0.58935546875;0.591796875;0.59423828125;0.5966796875;0.59912109375;0.6015625;0.60400390625;0.6064453125;0.60888671875;0.611328125;0.61376953125;0.6162109375;0.61865234375;0.62109375;0.62353515625;0.6259765625;0.62841796875;0.630859375;0.6328125;0.63525390625;0.6376953125;0.64013671875;0.642578125;0.64501953125;0.6474609375;0.6494140625;0.65185546875;0.654296875;0.65673828125;0.65869140625;0.6611328125;0.66357421875;0.666015625;0.66796875;0.67041015625;0.6728515625;0.6748046875;0.67724609375;0.67919921875;0.681640625;0.68408203125;0.68603515625;0.6884765625;0.6904296875;0.69287109375;0.69482421875;0.697265625;0.69921875;0.70166015625;0.70361328125;0.7060546875;0.7080078125;0.71044921875;0.71240234375;0.71484375;0.716796875;0.71875;0.72119140625;0.72314453125;0.72509765625;0.7275390625;0.7294921875;0.7314453125;0.73388671875;0.73583984375;0.73779296875;0.73974609375;0.7421875;0.744140625;0.74609375;0.748046875;0.75;0.75244140625;0.75439453125;0.75634765625;0.75830078125;0.76025390625;0.76220703125;0.76416015625;0.76611328125;0.76806640625;0.77001953125;0.77197265625;0.77392578125;0.77587890625;0.77783203125;0.77978515625;0.78173828125;0.78369140625;0.78564453125;0.78759765625;0.78955078125;0.79150390625;0.79296875;0.794921875;0.796875;0.798828125;0.80078125;0.80224609375;0.80419921875;0.80615234375;0.80810546875 ...(+2575 chars)]\"), [1  512])"  InterpMethod=Flat  ExtrapMethod=Clip  DiagnosticForOutOfRangeInput=Error  SampleTime=1e-08  OutDataTypeStr=fixdt(1, 18, 11)
  Negate : UnaryMinus  SampleTime=1e-08
  PipelineRegister : Delay  DelayLength=double(1)  InitialCondition=0  SampleTime=1e-08
  Point25 : Constant  Value=0.25  OutDataTypeStr=fixdt(0, 18, 18)  SampleTime=1e-08
  Point50 : Constant  Value=0.5  OutDataTypeStr=fixdt(0, 18, 18)  SampleTime=1e-08
  Point75 : Constant  Value=0.75  OutDataTypeStr=fixdt(0, 18, 18)  SampleTime=1e-08
  Positive : DataTypeConversion  OutDataTypeStr=fixdt(1, 18, 11)  SampleTime=1e-08  SaturateOnIntegerOverflow=off  RndMeth=Floor
  QuadHandle1a : Switch  Criteria=u2 ~= 0  Threshold=double(0)  OutDataTypeStr=fixdt(1, 19, 18)  SampleTime=1e-08  SaturateOnIntegerOverflow=off  InputSameDT=off
  QuadHandle1b : Switch  Criteria=u2 ~= 0  Threshold=double(0)  OutDataTypeStr=fixdt(1, 19, 18)  SampleTime=1e-08  SaturateOnIntegerOverflow=off  InputSameDT=off
  QuadHandle2 : Switch  Criteria=u2 ~= 0  Threshold=double(0)  OutDataTypeStr=fixdt(0, 11, 11)  SampleTime=1e-08  InputSameDT=off
  RAMDelayBalance : hdlmdlgenlib/Buffer
      settings: SourceProductBaseCode=SL
  Saturation : Saturate  UpperLimit="fi(0,0,11,0,\"hex\",\"1ff\")"  LowerLimit="fi(0,0,11,0,\"hex\",\"000\")"  SampleTime=1e-08  OutDataTypeStr=fixdt(0, 11, 0)
  SignCorrected : Switch  Criteria=u2 ~= 0  Threshold=double(0)  OutDataTypeStr=fixdt(1, 18, 11)  SampleTime=1e-08  SaturateOnIntegerOverflow=off  InputSameDT=off
  Switch : Switch  Criteria=u2 ~= 0  Threshold=double(0)  OutDataTypeStr=fixdt(0, 11, 0)  SampleTime=1e-08  SaturateOnIntegerOverflow=off  InputSameDT=off
  delayMatch : Delay  DelayLength=double(1)  InitialCondition=0  SampleTime=1e-08
  dtc : DataTypeConversion  OutDataTypeStr=uint8  SampleTime=1e-08  SaturateOnIntegerOverflow=off  RndMeth=Floor
  insig : DataTypeConversion  OutDataTypeStr=fixdt(0, 11, 11)  SampleTime=1e-08  SaturateOnIntegerOverflow=off  RndMeth=Floor
  p25mA : Sum  Inputs=+-  AccumDataTypeStr=fixdt(1, 19, 18)  OutDataTypeStr=fixdt(1, 19, 18)  SampleTime=1e-08
  p75mA : Sum  Inputs=+-  AccumDataTypeStr=fixdt(1, 19, 18)  OutDataTypeStr=fixdt(1, 19, 18)  SampleTime=1e-08
  pow2switch : Constant  OutDataTypeStr=boolean  SampleTime=1e-08
  x : Outport  SampleTime=1e-08
  wires:
  dtc/1 -> RAMDelayBalance/1
  Amp25/1 -> QuadHandle1a/3
  Amp75/1 -> QuadHandle1b/1
  CastU16En1/1 -> CastU16En3/1
  CastU16En2/1 -> Switch/3, Saturation/1
  CastU16En3/1 -> CastU16En2/1
  GTEp75/1 -> QuadHandle1b/2, 1st or 4th Quad/2
  LTEp25/1 -> QuadHandle1a/2, 1st or 4th Quad/1
  LTEp50/1 -> QuadHandle2/2
  PipelineRegister/1 -> Positive/1, Negate/1
  Negate/1 -> SignCorrected/3
  Point25/1 -> p25mA/1, LTEp25/2, Amp25/2
  Point50/1 -> LTEp50/2
  Point75/1 -> p75mA/1, GTEp75/2, Amp75/2
  Positive/1 -> SignCorrected/1
  QuadHandle1a/1 -> QuadHandle2/1
  QuadHandle1b/1 -> QuadHandle2/3
  QuadHandle2/1 -> CastU16En1/1
  delayMatch/1 -> SignCorrected/2
  Saturation/1 -> Switch/1
  SignCorrected/1 -> x/1
  Switch/1 -> Look-Up Table/1
  insig/1 -> p75mA/2, p25mA/2, LTEp50/1, LTEp25/1, GTEp75/1, Amp75/1, Amp25/1
  p25mA/1 -> QuadHandle1a/1
  p75mA/1 -> QuadHandle1b/3
  pow2switch/1 -> Switch/2
  1st or 4th Quad/1 -> dtc/1
  In1/1 -> insig/1
  RAMDelayBalance/1 -> delayMatch/1
  Look-Up Table/1 -> PipelineRegister/1
